simulink model "untitled"  (R2016b)
settings: Solver=VariableStepAuto  StartTime=0.0  StopTime=40  RelTol=1e-3
settings Model: Creator=Milan Sas  LastModifiedBy=Milan Sas

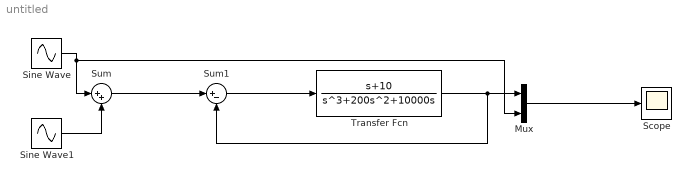
== system untitled ==
  Mux : Mux  Inputs=2
  Scope : Scope
  Sine Wave : Sin  Frequency=0.2  SampleTime=0
  Sine Wave1 : Sin  Frequency=2000  SampleTime=0
  Sum : Sum  Inputs=|++
  Sum1 : Sum  Inputs=|+-
  Transfer Fcn : TransferFcn  Numerator=[1 10]  Denominator=[1 200 10000 0]
  wires:
  Sine Wave/1 -> Mux/2, Sum/1
  Sine Wave1/1 -> Sum/2
  Sum/1 -> Sum1/1
  Mux/1 -> Scope/1
  Transfer Fcn/1 -> Sum1/2, Mux/1
  Sum1/1 -> Transfer Fcn/1
